simulink model "task_2_2"  (R2020b)
settings: Solver=VariableStepAuto  StartTime=0.0  StopTime=50  RelTol=1e-3
undefined symbols (not defined in the file): d_1, d_2, g, L, m_c, m_p
settings Model: Creator=rajag  LastModifiedBy=rajag

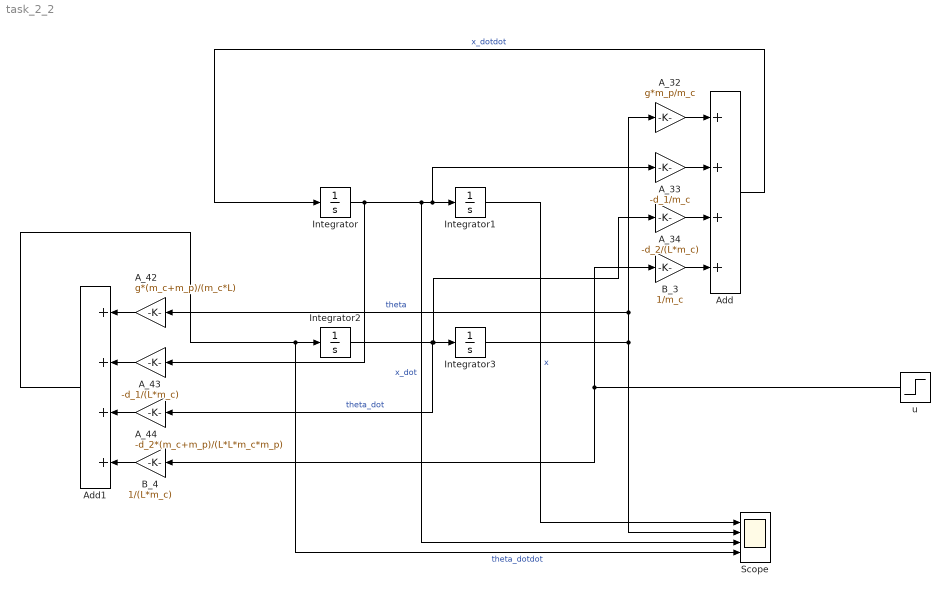
== system task_2_2 ==
  A_32 : Gain  Gain=g*m_p/m_c
  A_33 : Gain  Gain=-d_1/m_c
  A_34 : Gain  Gain=-d_2/(L*m_c)
  A_42 : Gain  Gain=g*(m_c+m_p)/(m_c*L)
  A_43 : Gain  Gain=-d_1/(L*m_c)
  A_44 : Gain  Gain=-d_2*(m_c+m_p)/(L*L*m_c*m_p)
  Add : Sum  Inputs=++++
  Add1 : Sum  Inputs=++++
  B_3 : Gain  Gain=1/m_c
  B_4 : Gain  Gain=1/(L*m_c)
  Integrator{,1..3} (4 alike) : Integrator
  Scope : Scope  NumInputPorts=4
  u : Step  SampleTime=0
  wires:
  Integrator/1 -> A_43/1, Scope/3, A_33/1, Integrator1/1  "x_dot"
  Add/1 -> Integrator/1  "x_dotdot"
  Integrator1/1 -> Scope/1  "x"
  Integrator3/1 -> Scope/2, A_42/1, A_32/1  "theta"
  Integrator2/1 -> A_44/1, A_34/1, Integrator3/1  "theta_dot"
  Add1/1 -> Scope/4, Integrator2/1  "theta_dotdot"
  A_32/1 -> Add/1
  A_33/1 -> Add/2
  A_34/1 -> Add/3
  B_3/1 -> Add/4
  u/1 -> B_4/1, B_3/1
  A_42/1 -> Add1/1
  B_4/1 -> Add1/4
  A_44/1 -> Add1/3
  A_43/1 -> Add1/2
